simulink model "Copy_of_Single_Phase_SAPF_02apr"  (R2017a)
settings: Solver=ode45  StartTime=0.0  StopTime=12  RelTol=1e-3  EnableMultiTasking=on
libraries: powerlib x24, powerlib_meascontrol x1, simulink_extras x1, simulink x1
settings Model: Creator=Niranjan  LastModifiedBy=Dell
settings DataIOCC: LimitDataPoints=on  SaveFormat=Array
settings OptimizationCC: LifeSpan=inf
settings DebuggingCC: SolverPrmCheckMsg=warning  SFUnexpectedBacktrackingDiag=warning  SFNoUnconditionalDefaultTransitionDiag=warning  SFExecutionAtInitializationDiag=none
settings HardwareCC: ProdBitPerPointer=32  ProdBitPerSizeT=32  ProdBitPerPtrDiffT=32  ProdLargestAtomicFloat=None  ProdIntDivRoundTo=Undefined  ProdEndianess=Unspecified  ProdWordSize=32  ProdHWDeviceType=32-bit Generic
settings ModelReferenceCC: PropagateSignalLabelsOutOfModel=off
settings GRTTargetCC: TargetLangStandard=C89/C90 (ANSI)  GeneratePreprocessorConditionals=Disable all
settings ConfigComp: CovMetricSettings=dw  CovHtmlReporting=on  CovSaveCumulativeToWorkspaceVar=on  CovSaveSingleToWorkspaceVar=on  CovExternalEMLEnable=off  CovSFcnEnable=off

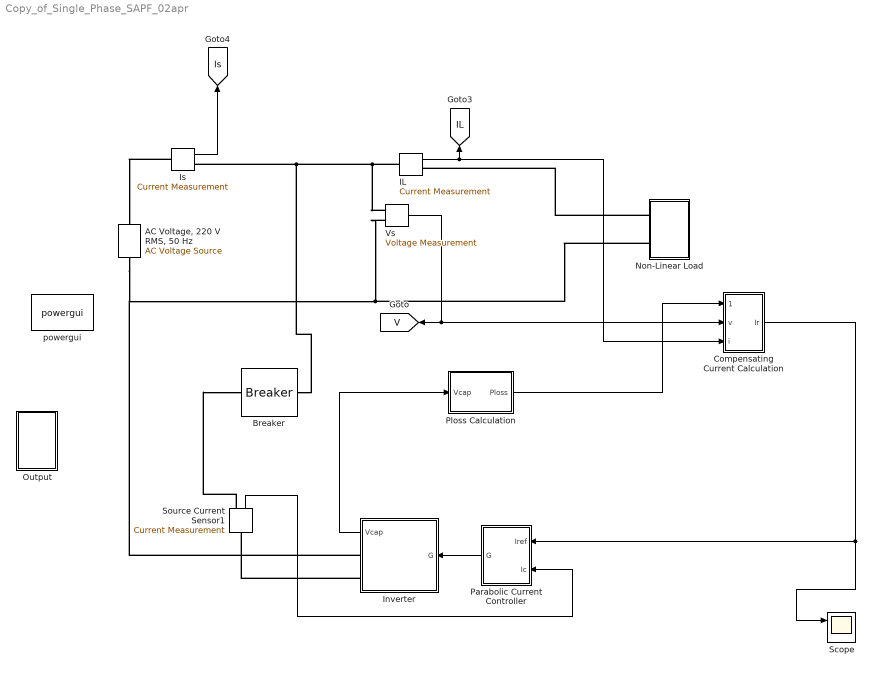
== system Copy_of_Single_Phase_SAPF_02apr ==
  "AC Voltage, 220 V RMS, 50 Hz" : powerlib/Electrical Sources/AC Voltage Source  Amplitude=311.13  Phase=0  Frequency=50  SampleTime=0  Measurements=None  BusType=swing  Pref=10e3  Qref=0  Qmin=-inf  Qmax=+inf
  Breaker : powerlib/Elements/Breaker  InitialState=0  SwitchingTimes=[0.965]  External=off  BreakerResistance=0.01  SnubberResistance=1e6  SnubberCapacitance=inf  Measurements=None  MoreParameters=on  NoBreakLoop=off
      settings: SourceProductName=Simscape Power Systems
  Compensating Current Calculation : Subsystem
  IL : powerlib/Measurements/Current Measurement  PhasorSimulation=off  OutputType=Complex  PSBequivalent=0
  Inverter : Subsystem
  Is : powerlib/Measurements/Current Measurement  PhasorSimulation=off  OutputType=Complex  PSBequivalent=0
  Non-Linear Load : Subsystem
  Output : Subsystem
  Parabolic Current Controller : Subsystem
  Ploss Calculation : Subsystem
  Scope : Scope  NumInputPorts=2
  Source Current Sensor1 : powerlib/Measurements/Current Measurement  PhasorSimulation=off  OutputType=Complex  PSBequivalent=0
  Vs : powerlib/Measurements/Voltage Measurement  PhasorSimulation=off  OutputType=Complex  PSBequivalent=0
  powergui : powerlib/powergui  Priority=1  SimulationMode=Discrete  SampleTime=1e-4  frequency=60  Iterations=50  frequencyindice=50  Pbase=100e6  ErrMax=1e-4  UnitsV=kV  UnitsW=MW  buscounter=0  FunctionMessages=off  echomessages=off  EnableUseOfTLC=off  CurrentSourceSwitches=off  DisableSnubberDevices=off  DisableRonSwitches=off  DisableVfSwitches=off  DisplayEquations=off  SolverType=Tustin/Backward Euler (TBE)  Interpol=off  ExternalGateDelay=off  methode=off  Ts=10  x0status=blocks  SPID=off  SwTol=0  HookPort=off  RestoreLinks=warning  ResistiveCurrentMeasurement=off  Frange=[0:2:500]  Ylog=off  Xlog=on  ShowGrid=off  save=off  variable=ZData  structure=ScopeData_PCC  ZoomFFT=off  StartTime=1.2  cycles=1  DisplayStyle=1  fundamental=50  FreqAxis=on  MaxFrequency=3000  frequencyindicesteady=1  RmsSteady=1  display=off
  tag scope: IL=global, Is=global, V=global
  wires:
  IL/1 -> Compensating Current Calculation/3(i), [IL]
  Vs/1 -> Compensating Current Calculation/2(v), [V]
  Is/1 -> [Is]
  Source Current Sensor1/1 -> Parabolic Current Controller/2(Ic)
  Parabolic Current Controller/1(G) -> Inverter/1(G)
  Inverter/1(Vcap) -> Ploss Calculation/1(Vcap)
  Ploss Calculation/1(Ploss) -> Compensating Current Calculation/1(Ploss)
  Compensating Current Calculation/1(Ir) -> Parabolic Current Controller/1(Iref), Scope/1
  connections:
  Is/LConn1 -- "AC Voltage, 220 V RMS, 50 Hz"/RConn1
  Non-Linear Load/LConn1 -- IL/RConn1
  Inverter/RConn1 -- "AC Voltage, 220 V RMS, 50 Hz"/LConn1 -- Vs/LConn2 -- Non-Linear Load/LConn2
  Inverter/RConn2 -- Source Current Sensor1/LConn1
  IL/LConn1 -- Breaker/RConn1 -- Is/RConn1 -- Vs/LConn1
  Source Current Sensor1/RConn1 -- Breaker/LConn1

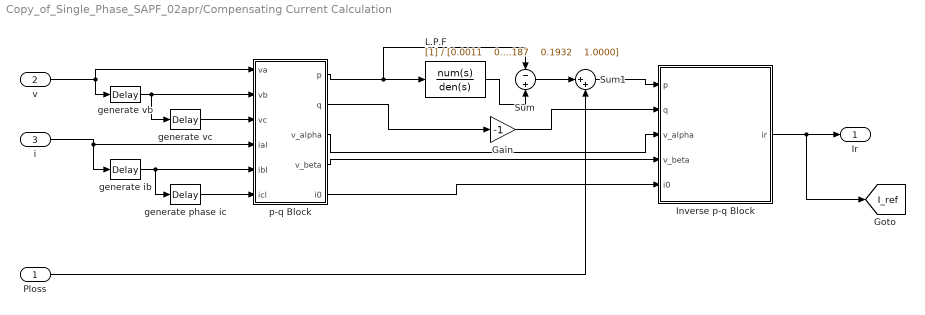
== system Copy_of_Single_Phase_SAPF_02apr/Compensating Current Calculation ==
  Ploss : Inport
  v : Inport  Port=2
  i : Inport  Port=3
  Gain : Gain  Gain=-1
  Inverse p-q Block : MATLAB Function  TreatAsAtomicUnit=on
  L.P.F : TransferFcn  Denominator="[0.0011    0.0187    0.1932    1.0000]"
  Sum : Sum  Inputs=-+
  Sum1 : Sum  Inputs=|++
  generate phase ic : TransportDelay  DelayTime=1/150  BufferSize=10240
  generate ib : TransportDelay  DelayTime=1/150  BufferSize=10240
  generate vb : TransportDelay  DelayTime=1/150  BufferSize=10240
  generate vc : TransportDelay  DelayTime=1/150  BufferSize=10240
  p-q Block : MATLAB Function  TreatAsAtomicUnit=on
  Ir : Outport
  tag scope: I_ref=global
  wires:
  p-q Block/1(p) -> Sum/1, L.P.F/1
  Ploss/1 -> Sum1/2
  Sum/1 -> Sum1/1
  Sum1/1 -> Inverse p-q Block/1(p)
  v/1 -> generate vb/1, p-q Block/1(va)
  i/1 -> generate ib/1, p-q Block/4(ial)
  generate vb/1 -> generate vc/1, p-q Block/2(vb)
  generate vc/1 -> p-q Block/3(vc)
  generate ib/1 -> generate phase ic/1, p-q Block/5(ibl)
  generate phase ic/1 -> p-q Block/6(icl)
  p-q Block/3(v_alpha) -> Inverse p-q Block/3(v_alpha)
  p-q Block/4(v_beta) -> Inverse p-q Block/4(v_beta)
  L.P.F/1 -> Sum/2
  p-q Block/5(i0) -> Inverse p-q Block/5(i0)
  Inverse p-q Block/1(ir) -> [I_ref], Ir/1
  p-q Block/2(q) -> Gain/1
  Gain/1 -> Inverse p-q Block/2(q)

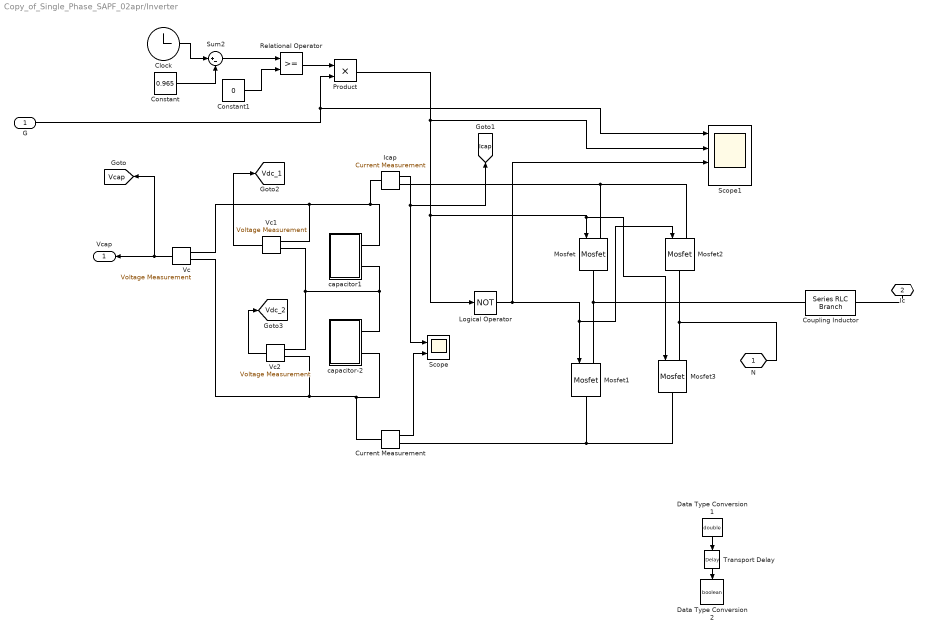
== system Copy_of_Single_Phase_SAPF_02apr/Inverter ==
  G : Inport
  Clock : Clock
  Constant : Constant  Value=0.965
  Constant1 : Constant  Value=0
  Coupling Inductor : powerlib/Elements/Series RLC Branch  LConnTagsString=__new0  RConnTagsString=__new0  BranchType=RL  Resistance=0.1  Inductance=15e-3  SetiL0=off  InitialCurrent=0  Capacitance=0.015  Setx0=off  InitialVoltage=0  Measurements=None
  Current Measurement : powerlib/Measurements/Current Measurement  PhasorSimulation=off  OutputType=Complex  PSBequivalent=0
  Data Type Conversion1 : DataTypeConversion  OutDataTypeStr=double
  Data Type Conversion2 : DataTypeConversion  OutDataTypeStr=boolean
  Icap : powerlib/Measurements/Current Measurement  PhasorSimulation=off  OutputType=Complex  PSBequivalent=0
  Logical Operator : Logic  Operator=NOT  IconShape=distinctive  AllPortsSameDT=off  OutDataTypeStr=boolean
  Mosfet{,1..3} (4 alike) : powerlib/Power Electronics/Mosfet  Ron=0.1  Lon=0  Rd=0.01  Vfd=0  IC=0  Rs=1e5  Cs=inf  Measurements=off
  Product : Product
  Relational Operator : RelationalOperator  OutDataTypeStr=boolean  RndMeth=Simplest
  Scope : Scope  NumInputPorts=2
  Scope1 : Scope  NumInputPorts=4
  Sum2 : Sum  Inputs=|+-
  Transport Delay : TransportDelay  DelayTime=2e-6
  Vc : powerlib/Measurements/Voltage Measurement  PhasorSimulation=off  OutputType=Complex  PSBequivalent=0
  Vc1 : powerlib/Measurements/Voltage Measurement  PhasorSimulation=off  OutputType=Complex  PSBequivalent=0
  Vc2 : powerlib/Measurements/Voltage Measurement  PhasorSimulation=off  OutputType=Complex  PSBequivalent=0
  capacitor-2 : Subsystem
  capacitor1 : Subsystem
  N : PMIOPort  Port=1  Side=Right
  Ic : PMIOPort  Port=2  Side=Right
  Vcap : Outport
  tag scope: Icap=global, Vcap=global, Vdc_1=global, Vdc_2=global
  wires:
  Vc/1 -> [Vcap], Vcap/1
  Icap/1 -> Scope/1, [Icap]
  Current Measurement/1 -> Scope/2
  Data Type Conversion1/1 -> Transport Delay/1
  Transport Delay/1 -> Data Type Conversion2/1
  Sum2/1 -> Relational Operator/1
  Clock/1 -> Sum2/1
  Constant/1 -> Sum2/2
  Constant1/1 -> Relational Operator/2
  Relational Operator/1 -> Product/1
  G/1 -> Scope1/1, Product/2
  Logical Operator/1 -> Scope1/3, Mosfet2/1, Mosfet1/1
  Product/1 -> Logical Operator/1, Mosfet3/1, Mosfet/1, Scope1/2
  Vc1/1 -> [Vdc_1]
  Vc2/1 -> [Vdc_2]
  connections:
  Mosfet1/LConn1 -- Coupling Inductor/RConn1 -- Mosfet/RConn1
  capacitor-2/RConn2 -- Vc2/LConn2 -- Vc/LConn2 -- Current Measurement/LConn1
  Icap/LConn1 -- capacitor1/RConn1 -- Vc1/LConn1 -- Vc/LConn1
  Coupling Inductor/LConn1 -- Ic/RConn1
  Mosfet1/RConn1 -- Mosfet3/RConn1 -- Current Measurement/RConn1
  Mosfet/LConn1 -- Mosfet2/LConn1 -- Icap/RConn1
  capacitor-2/RConn1 -- Vc1/LConn2 -- Vc2/LConn1 -- capacitor1/RConn2
  Mosfet3/LConn1 -- N/RConn1 -- Mosfet2/RConn1

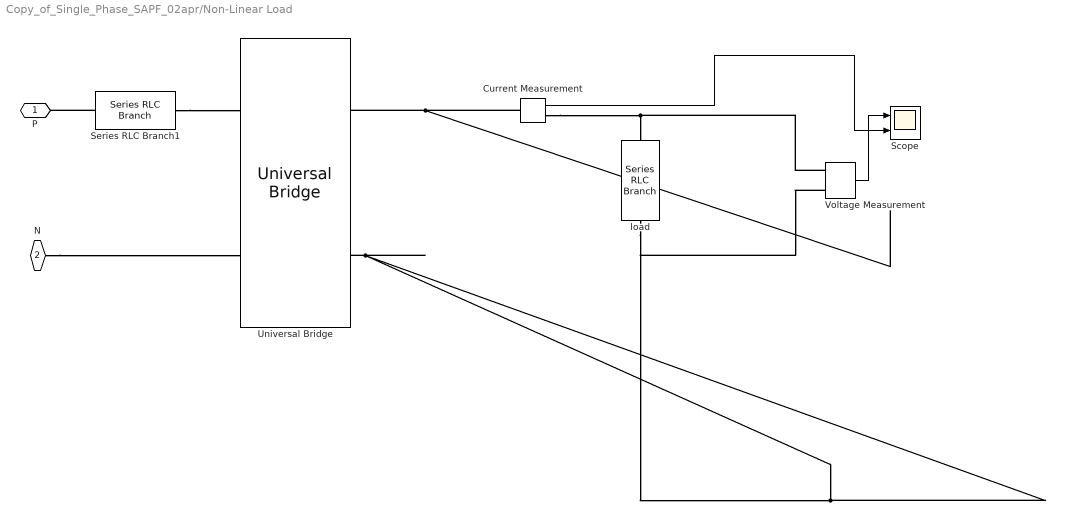
== system Copy_of_Single_Phase_SAPF_02apr/Non-Linear Load ==
  " load" : powerlib/Elements/Series RLC Branch  LConnTagsString=__new0  RConnTagsString=__new0  BranchType=R  Resistance=100  Inductance=1e-3  SetiL0=off  InitialCurrent=0  Capacitance=0.015  Setx0=off  InitialVoltage=0  Measurements=None
  Current Measurement : powerlib/Measurements/Current Measurement  PhasorSimulation=off  OutputType=Complex  PSBequivalent=0
  Scope : Scope  NumInputPorts=2
  Series RLC Branch1 : powerlib/Elements/Series RLC Branch  LConnTagsString=__new0  RConnTagsString=__new0  BranchType=L  Resistance=1  Inductance=2e-3  SetiL0=on  InitialCurrent=3  Capacitance=1e-6  Setx0=off  InitialVoltage=0  Measurements=None
  Universal Bridge : powerlib/Power Electronics/Universal Bridge  Arms=2  SnubberResistance=1e5  SnubberCapacitance=inf  Device=Diodes  Ron=1e-3  Lon=0  ForwardVoltages="[  0  0  ]"  ForwardVoltage=0  GTOparameters=[ 10e-6 , 20e-6 ]  IGBTparameters=[ 1e-6 , 2e-6 ]  Measurements=None  Measurements_2=None  converterType=Rectifier
  Voltage Measurement : powerlib/Measurements/Voltage Measurement  PhasorSimulation=off  OutputType=Complex  PSBequivalent=0
  P : PMIOPort  Port=1  Side=Left
  N : PMIOPort  Port=2  Side=Left
  wires:
  Voltage Measurement/1 -> Scope/1
  Current Measurement/1 -> Scope/2
  connections:
  Current Measurement/RConn1 -- Voltage Measurement/LConn1 -- " load"/LConn1
  Universal Bridge/RConn2 -- Voltage Measurement/LConn2 -- " load"/RConn1
  Current Measurement/LConn1 -- Universal Bridge/RConn1
  N/RConn1 -- Universal Bridge/LConn2
  Series RLC Branch1/RConn1 -- Universal Bridge/LConn1
  Series RLC Branch1/LConn1 -- P/RConn1

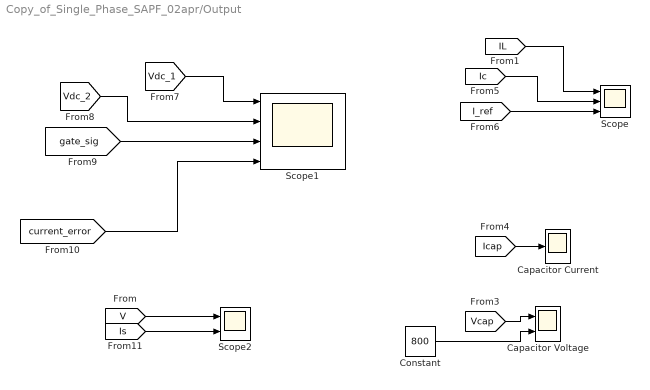
== system Copy_of_Single_Phase_SAPF_02apr/Output ==
  Capacitor Current : Scope
  Capacitor Voltage : Scope  NumInputPorts=2
  Constant : Constant  Value=800
  Scope : Scope  NumInputPorts=3
  Scope1 : Scope  NumInputPorts=4
  Scope2 : Scope  NumInputPorts=2
  wires:
  [Vcap] -> Capacitor Voltage/1
  [Icap] -> Capacitor Current/1
  [I_ref] -> Scope/3
  [IL] -> Scope/1
  Constant/1 -> Capacitor Voltage/2
  [Vdc_1] -> Scope1/1
  [Vdc_2] -> Scope1/2
  [gate_sig] -> Scope1/3
  [current_error] -> Scope1/4
  [Ic] -> Scope/2
  [V] -> Scope2/1
  [Is] -> Scope2/2

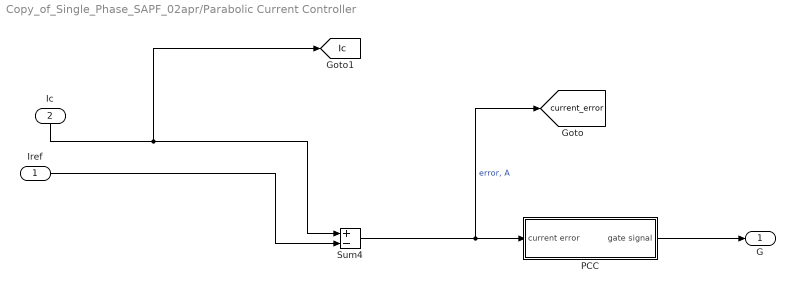
== system Copy_of_Single_Phase_SAPF_02apr/Parabolic Current Controller ==
  Iref : Inport
  Ic : Inport  Port=2
  "PCC " : Subsystem
  Sum4 : Sum  Inputs=+-
  G : Outport
  tag scope: Ic=global, current_error=global
  wires:
  "PCC "/1(gate signal) -> G/1
  Iref/1 -> Sum4/2
  Ic/1 -> Sum4/1, [Ic]
  Sum4/1 -> "PCC "/1(current error), [current_error]  "error, A"

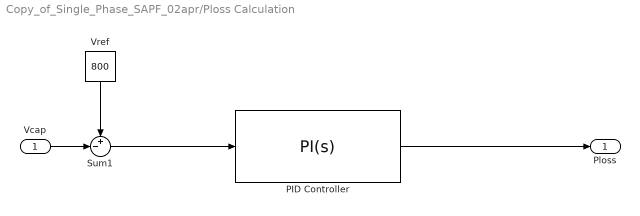
== system Copy_of_Single_Phase_SAPF_02apr/Ploss Calculation ==
  Vcap : Inport
  PID Controller : simulink/Continuous/PID Controller  Controller=PI  TimeDomain=Continuous-time  SampleTime=-1  IntegratorMethod=Forward Euler  FilterMethod=Forward Euler  Form=Parallel  UseFilter=on  ControllerParametersSource=internal  P=5  I=1200  D=0  N=100  InitialConditionSource=internal  InitialConditionForIntegrator=0  InitialConditionForFilter=0  ExternalReset=none  LimitOutput=on  UpperSaturationLimit=1e6  LowerSaturationLimit=-1e6  LinearizeAsGain=on  AntiWindupMode=clamping  Kb=1  TrackingMode=off  Kt=1  PParamMin=[]  PParamMax=[]  IParamMin=[]  IParamMax=[]  DParamMin=[]  DParamMax=[]  NParamMin=[]  NParamMax=[]  KbParamMin=[]  KbParamMax=[]  KtParamMin=[]  KtParamMax=[]  POutMin=[]  POutMax=[]  IOutMin=[]  IOutMax=[]  DOutMin=[]  DOutMax=[]  NOutMin=[]  NOutMax=[]  KbOutMin=[]  KbOutMax=[]  KtOutMin=[]  KtOutMax=[]  IntegratorOutMin=[]  IntegratorOutMax=[]  FilterOutMin=[]  FilterOutMax=[]  SumOutMin=[]  SumOutMax=[]  SumI1OutMin=[]  SumI1OutMax=[]  SumI2OutMin=[]  SumI2OutMax=[]  SumI3OutMin=[]  SumI3OutMax=[]  SumDOutMin=[]  SumDOutMax=[]  SaturationOutMin=[]  SaturationOutMax=[]  IntegratorContinuousStateAttributes=''  IntegratorStateMustResolveToSignalObject=off  IntegratorRTWStateStorageClass=Auto  FilterContinuousStateAttributes=''  FilterStateMustResolveToSignalObject=off  FilterRTWStateStorageClass=Auto  DifferentiatorICPrevScaledInput=0  DifferentiatorOutMin=[]  DifferentiatorOutMax=[]  InitialConditionSetting=State (most efficient)
  Sum1 : Sum  Inputs=+-|
  Vref : Constant  Value=800
  Ploss : Outport
  wires:
  Vcap/1 -> Sum1/2
  Vref/1 -> Sum1/1
  PID Controller/1 -> Ploss/1
  Sum1/1 -> PID Controller/1

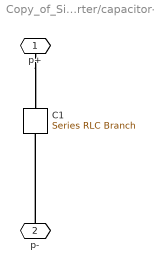
== system Copy_of_Single_Phase_SAPF_02apr/Inverter/capacitor-2 ==
  "C1 " : powerlib/Elements/Series RLC Branch  LConnTagsString=__new0  RConnTagsString=__new0  BranchType=C  Resistance=1e-9  Inductance=1e-9  SetiL0=off  InitialCurrent=0  Capacitance=3000e-6  Setx0=on  InitialVoltage=420  Measurements=None
  p+ : PMIOPort  Port=1  Side=Right
  p- : PMIOPort  Port=2  Side=Right
  connections:
  p-/RConn1 -- "C1 "/RConn1
  p+/RConn1 -- "C1 "/LConn1

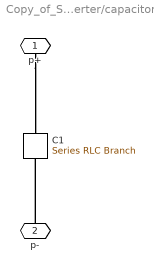
== system Copy_of_Single_Phase_SAPF_02apr/Inverter/capacitor1 ==
  "C1 " : powerlib/Elements/Series RLC Branch  LConnTagsString=__new0  RConnTagsString=__new0  BranchType=C  Resistance=1e-9  Inductance=1e-9  SetiL0=off  InitialCurrent=0  Capacitance=3000e-6  Setx0=on  InitialVoltage=420  Measurements=None
  p+ : PMIOPort  Port=1  Side=Right
  p- : PMIOPort  Port=2  Side=Right
  connections:
  p-/RConn1 -- "C1 "/RConn1
  p+/RConn1 -- "C1 "/LConn1

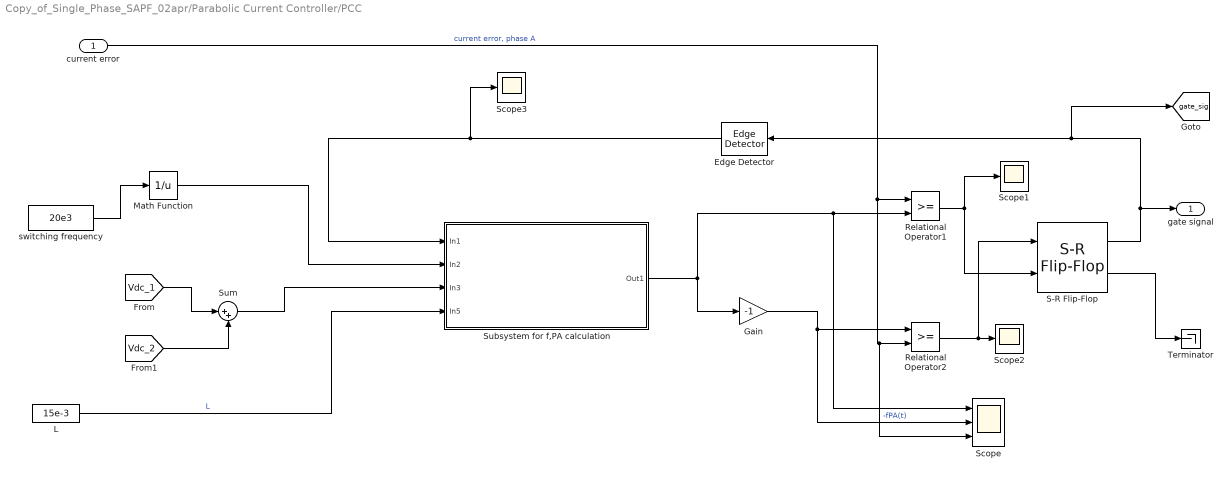
== system Copy_of_Single_Phase_SAPF_02apr/Parabolic Current Controller/PCC  ==
  current error : Inport
  Edge Detector : powerlib_meascontrol/Logic/Edge Detector  model=Either  ic=0  Ts=0
      settings: SourceProductName=Simscape Power Systems  SourceProductBaseCode=PS
  Gain : Gain  Gain=-1
  L : Constant  Value=15e-3
  Math Function : Math  Operator=reciprocal  SaturateOnIntegerOverflow=on
  Relational Operator1 : RelationalOperator  OutDataTypeStr=boolean  ZeroCross=off  RndMeth=Simplest
  Relational Operator2 : RelationalOperator  OutDataTypeStr=boolean  ZeroCross=off  RndMeth=Simplest
  S-R Flip-Flop : simulink_extras/Flip Flops/S-R Flip-Flop  initial_condition=1
  Scope : Scope  NumInputPorts=3
  Scope1 : Scope
  Scope2 : Scope
  Scope3 : Scope
  Subsystem for f,PA calculation : Subsystem
  Sum : Sum  Inputs=|++
  Terminator : Terminator
  switching frequency : Constant  Value=20e3
  gate signal : Outport
  tag scope: gate_sig=global
  wires:
  current error/1 -> Relational Operator1/1, Scope/3, Relational Operator2/2  "current error, phase A"
  S-R Flip-Flop/1 -> [gate_sig], Edge Detector/1, gate signal/1
  Relational Operator1/1 -> S-R Flip-Flop/2, Scope1/1
  Relational Operator2/1 -> S-R Flip-Flop/1, Scope2/1
  S-R Flip-Flop/2 -> Terminator/1
  Subsystem for f,PA calculation/1(Out1) -> Scope/1, Relational Operator1/2, Gain/1
  Gain/1 -> Scope/2, Relational Operator2/1  "-fPA(t)"
  Edge Detector/1 -> Scope3/1, Subsystem for f,PA calculation/1(In1)
  switching frequency/1 -> Math Function/1
  L/1 -> Subsystem for f,PA calculation/4(In5)  "L"
  Math Function/1 -> Subsystem for f,PA calculation/2(In2)
  Sum/1 -> Subsystem for f,PA calculation/3(In3)
  [Vdc_1] -> Sum/1
  [Vdc_2] -> Sum/2

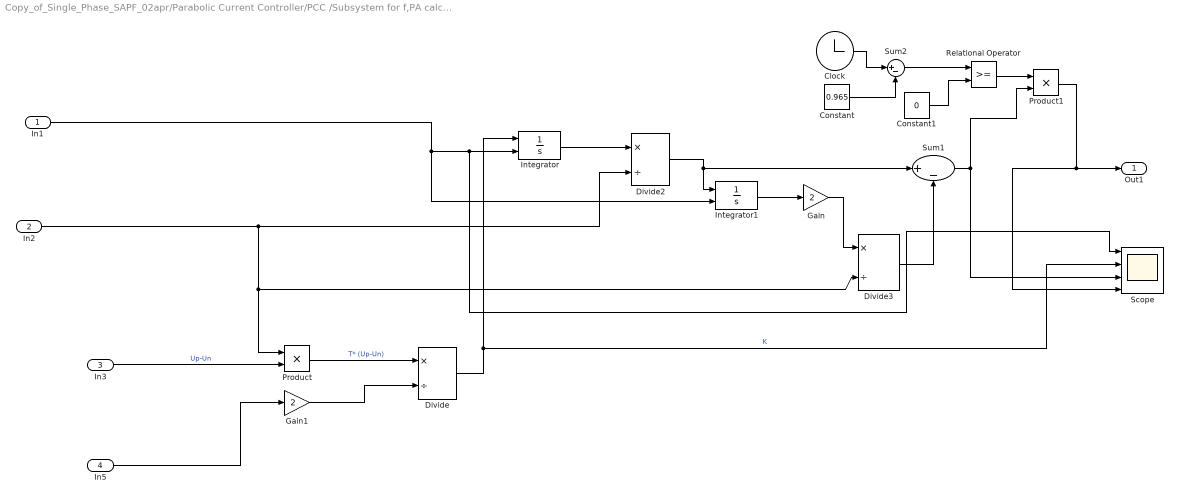
== system Copy_of_Single_Phase_SAPF_02apr/Parabolic Current Controller/PCC /Subsystem for f,PA calculation ==
  In1 : Inport
  In2 : Inport  Port=2
  In3 : Inport  Port=3
  In5 : Inport  Port=4
  Clock : Clock
  Constant : Constant  Value=0.965
  Constant1 : Constant  Value=0
  Divide : Product  Inputs=*/
  Divide2 : Product  Inputs=*/
  Divide3 : Product  Inputs=*/
  Gain : Gain  Gain=2
  Gain1 : Gain  Gain=2
  Integrator : Integrator  ExternalReset=either
  Integrator1 : Integrator  ExternalReset=either
  Product : Product
  Product1 : Product
  Relational Operator : RelationalOperator  OutDataTypeStr=boolean  RndMeth=Simplest
  Scope : Scope  NumInputPorts=4
  Sum1 : Sum  Inputs=|+-
  Sum2 : Sum  Inputs=|+-
  Out1 : Outport
  wires:
  In5/1 -> Gain1/1
  Gain1/1 -> Divide/2
  Divide3/1 -> Sum1/2
  In3/1 -> Product/2  "Up-Un"
  Product/1 -> Divide/1  "T* (Up-Un)"
  In1/1 -> Integrator1/2, Scope/1, Integrator/2
  Integrator1/1 -> Gain/1
  In2/1 -> Product/1, Divide3/2, Divide2/2
  Divide/1 -> Integrator/1, Scope/2  "K"
  Integrator/1 -> Divide2/1
  Divide2/1 -> Sum1/1, Integrator1/1
  Gain/1 -> Divide3/1
  Clock/1 -> Sum2/1
  Sum1/1 -> Product1/2, Scope/3
  Constant1/1 -> Relational Operator/2
  Constant/1 -> Sum2/2
  Relational Operator/1 -> Product1/1
  Sum2/1 -> Relational Operator/1
  Product1/1 -> Out1/1, Scope/4

== matlab function Copy_of_Single_Phase_SAPF_02apr/Compensating Current Calculation/Inverse p-q Block ==
  data: p input; q input; v_alpha input; v_beta input; ir output; i0 input
function ir = fcn(p,q,v_alpha,v_beta,i0)
%#codegen
i_alpha=(v_alpha.*p+v_beta.*q)/(v_alpha.^2+v_beta.^2);
i_beta=(v_beta.*p-v_alpha.*q)/(v_alpha.^2+v_beta.^2);
ir=sqrt(2/3)*(i0/sqrt(2)+i_alpha);

== matlab function Copy_of_Single_Phase_SAPF_02apr/Compensating Current Calculation/p-q Block ==
  data: va input; p output; vb input; vc input; ial input; ibl input; icl input; q output; v_alpha output; v_beta output; i0 output
function [p,q,v_alpha,v_beta,i0]= fcn(va,vb,vc,ial,ibl,icl)
%#codegen
v_alpha=(va-vb/2-vc/2)*sqrt(2/3);
v_beta=(vb-vc)/sqrt(2);
i0=(ial+ibl+icl)/sqrt(3);
il_alpha=(ial-ibl/2-icl/2)*sqrt(2/3);
il_beta=(ibl-icl)/sqrt(2);
p=v_alpha.*il_alpha+v_beta.*il_beta;
q=v_beta.*il_alpha-v_alpha.*il_beta;
